simulink model "simple_system_sim"  (R2022a)
settings: Solver=ode45  StartTime=0.0  StopTime=15.0  RelTol=1e-3
values from neighbouring files (symbols this model uses):
  J = 1/4*m*R^2+1/3*m*l^2    (= 0.333958333333)    [simple_system.m]
  Kpp = wcp    (= 31.4159265359)    [simple_system.m]
  Kpv = wcv/mu    (= 104.916104661)    [simple_system.m]
  L = 30    [simple_system.m]
  l = 1.0    (= 1)    [simple_system.m]
  m = 1.0    (= 1)    [simple_system.m]
  Tff = 1/(wff*2*pi)    (= 0.00318309886184)    [simple_system.m]
  Tiv = 1/(0.1*wcv)    (= 0.0318309886184)    [simple_system.m]
  Tlpf = 1/(wlpf*2*pi)    (= 0.0318309886184)    [simple_system.m]
libraries: simulink x6
settings Model: Creator=ale  LastModifiedBy=ale

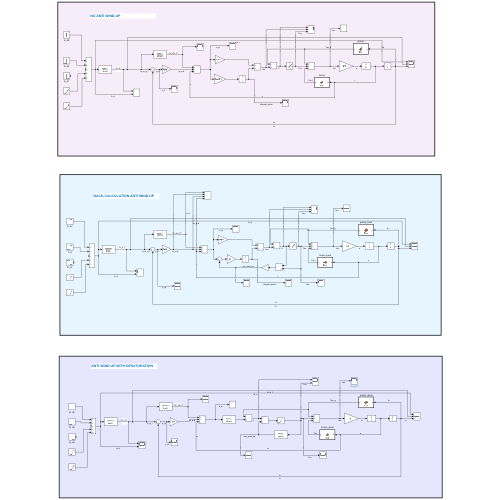
[thumbnail: Simulink's stored preview of the top-level diagram]
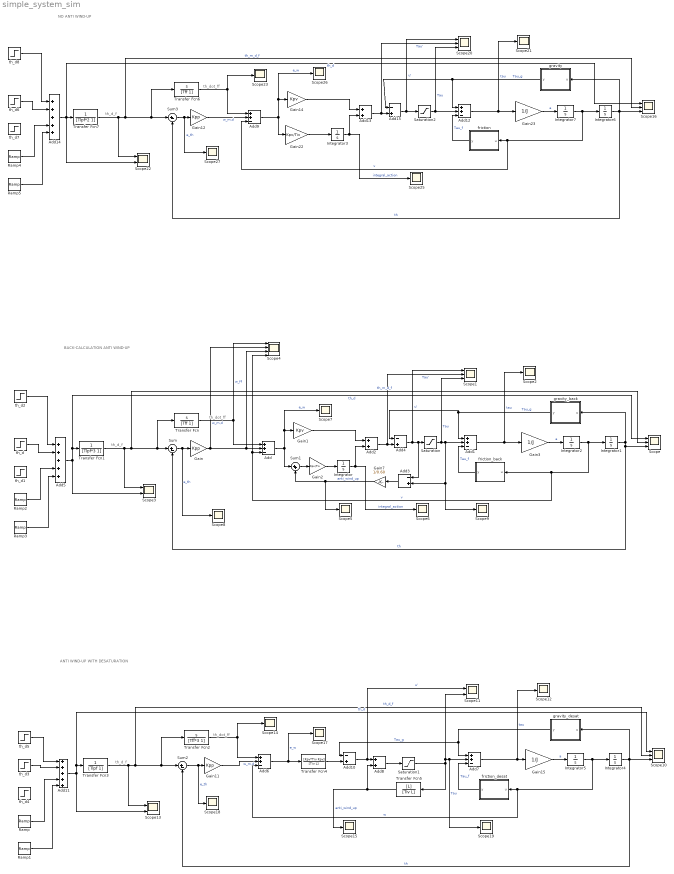
== system simple_system_sim ==
  note: BACK-CALCULATION ANTI WIND-UP
  note: th_dot_ff
  note: th_d_f
  note: th_dot_ff
  note: th_d_f
  note: ANTI WIND-UP WITH DESATURATION
  note: th_d_f
  note: th_dot_ff
  note: NO ANTI WIND-UP
  Add{,1,6..7,9,12} (6 alike) : Sum  Inputs=++-
  Add{3..4,10,15} (4 alike) : Sum  Inputs=-+
  Add11 : Sum  Inputs=+++++
  Add13 : Sum
  Add14 : Sum  Inputs=+++++
  Add2 : Sum
  Add5 : Sum  Inputs=+++++
  Add8 : Sum
  Gain : Gain  Gain=Kpp
  Gain1 : Gain  Gain=Kpv
  Gain11 : Gain  Gain=Kpp
  Gain12 : Gain  Gain=Kpp
  Gain14 : Gain  Gain=Kpv
  Gain15 : Gain  Gain=1/J
  Gain2 : Gain  Gain=Kpv/Tiv
  Gain22 : Gain  Gain=Kpv/Tiv
  Gain23 : Gain  Gain=1/J
  Gain3 : Gain  Gain=1/J
  Gain7 : Gain  Gain=1/0.60
  Integrator{,1..7} (8 alike) : Integrator
  Ramp : simulink/Sources/Ramp  slope=-pi/2  start=6  InitialOutput=0
  Ramp1 : simulink/Sources/Ramp  slope=+pi/2  start=7  InitialOutput=0
  Ramp2 : simulink/Sources/Ramp  slope=-pi/2  start=6  InitialOutput=0
  Ramp3 : simulink/Sources/Ramp  slope=+pi/2  start=7  InitialOutput=0
  Ramp4 : simulink/Sources/Ramp  slope=-pi/2  start=6  InitialOutput=0
  Ramp5 : simulink/Sources/Ramp  slope=+pi/2  start=7  InitialOutput=0
  Saturation : Saturate  UpperLimit=6  LowerLimit=-6
  Saturation1 : Saturate  UpperLimit=6  LowerLimit=-6
  Saturation2 : Saturate  UpperLimit=6  LowerLimit=-6
  Scope{,1,10,16,20} (5 alike) : Scope  NumInputPorts=3
  Scope{3,11,13,22} (4 alike) : Scope  NumInputPorts=2
  Scope{2,5..9,12,14..15,17..19,21,23,25..27} (17 alike) : Scope
  Scope4 : Scope  NumInputPorts=4
  Sum : Sum  Inputs=|+-
  Sum1 : Sum  Inputs=|++
  Sum2 : Sum  Inputs=|+-
  Sum3 : Sum  Inputs=|+-
  Transfer Fcn : TransferFcn  Numerator=[1 0]  Denominator=[Tff 1]
  Transfer Fcn1 : TransferFcn  Denominator=[Tlpf*3 1]
  Transfer Fcn2 : TransferFcn  Numerator=[1 0]  Denominator=[Tff*3 1]
  Transfer Fcn3 : TransferFcn  Denominator=[Tlpf 1]
  Transfer Fcn4 : TransferFcn  Numerator=[Kpv*Tiv Kpv]  Denominator=[Tiv L]
  Transfer Fcn5 : TransferFcn  Numerator=[L]  Denominator=[Tiv L]
  Transfer Fcn6 : TransferFcn  Numerator=[1 0]  Denominator=[Tff 1]
  Transfer Fcn7 : TransferFcn  Denominator=[Tlpf*2 1]
  friction : MATLAB Function  TreatAsAtomicUnit=on
  friction_back : MATLAB Function  TreatAsAtomicUnit=on
  friction_desat : MATLAB Function  TreatAsAtomicUnit=on
  gravity : MATLAB Function  TreatAsAtomicUnit=on
  gravity_back : MATLAB Function  TreatAsAtomicUnit=on
  gravity_desat : MATLAB Function  TreatAsAtomicUnit=on
  th_d : Step  After=pi/18  SampleTime=0
  th_d1 : Step  Time=6  After=-pi/2  SampleTime=0
  th_d2 : Step  Time=3  After=pi/18  SampleTime=0
  th_d3 : Step  After=pi/18  SampleTime=0
  th_d4 : Step  Time=6  After=-pi/2  SampleTime=1
  th_d5 : Step  Time=3  After=pi/18  SampleTime=0
  th_d6 : Step  After=pi/18  SampleTime=0
  th_d7 : Step  Time=6  After=-pi/2  SampleTime=0
  th_d8 : Step  Time=3  After=pi/18  SampleTime=0
  wires:
  Sum/1 -> Gain/1, Scope8/1  "e_th"
  Gain1/1 -> Add2/1
  Integrator/1 -> Add2/2, Scope6/1  "integral_action"
  Add/1 -> Sum1/1, Gain1/1, Scope7/1  "e_w"
  Add2/1 -> Add4/2, Scope1/2  "Tau'"
  Integrator1/1 -> Sum/2, Scope/3, gravity_back/1(u)  "th"
  Gain3/1 -> Integrator2/1  "a"
  Integrator2/1 -> friction_back/1(u), Add/3, Scope4/4, Integrator1/1  "v"
  gravity_back/1(y) -> Add4/1, Add1/1  "Tau_g"
  Transfer Fcn1/1 -> Scope3/1, Transfer Fcn/1, Sum/1, Scope/2  "th_m_d_f"
  Saturation/1 -> Scope9/1, Add3/2, Add1/2, Scope1/3  "Tau"
  Add3/1 -> Gain7/1
  Gain7/1 -> Scope5/1, Sum1/2  "anti_wind_up"
  Add1/1 -> Gain3/1, Scope2/1  "tau"
  Transfer Fcn/1 -> Add/1, Scope4/1  "w_ff"
  Add4/1 -> Scope1/1, Add3/1, Saturation/1  "u'"
  Add5/1 -> Scope3/2, Scope/1, Transfer Fcn1/1  "th_d"
  th_d2/1 -> Add5/1
  th_d/1 -> Add5/2
  Integrator4/1 -> Sum2/2, Scope10/3, gravity_desat/1(u)  "th"
  gravity_desat/1(y) -> Add7/1, Add10/1  "Tau_g"
  Sum2/1 -> Scope18/1, Gain11/1  "e_th"
  Add11/1 -> Scope10/1, Transfer Fcn3/1, Scope13/2  "th_d"
  th_d5/1 -> Add11/1
  th_d3/1 -> Add11/2
  Gain15/1 -> Integrator5/1  "a"
  Add6/1 -> Transfer Fcn4/1, Scope17/1  "e_w"
  Transfer Fcn2/1 -> Scope14/1, Add6/1
  friction_desat/1(y) -> Add7/3  "Tau_f"
  Transfer Fcn3/1 -> Scope13/1, Transfer Fcn2/1, Sum2/1, Scope10/2  "th_d_f"
  Saturation1/1 -> Transfer Fcn5/1, Scope19/1, Add7/2, Scope11/2  "Tau"
  Gain11/1 -> Add6/2  "w_m,d"
  Transfer Fcn5/1 -> Add8/2, Scope15/1  "anti_wind_up"
  Integrator5/1 -> Add6/3, friction_desat/1(u), Integrator4/1  "w"
  Add7/1 -> Gain15/1, Scope12/1  "tau"
  Transfer Fcn4/1 -> Add10/2
  Add10/1 -> Scope11/1, Add8/1  "u'"
  Add8/1 -> Saturation1/1
  friction_back/1(y) -> Add1/3  "Tau_f"
  Saturation2/1 -> Add12/2, Scope20/3  "Tau"
  Add13/1 -> Add15/2, Scope20/2  "Tau'"
  Gain14/1 -> Add13/1
  Add14/1 -> Scope16/1, Scope22/2, Transfer Fcn7/1  "th_d"
  Gain12/1 -> Add9/2  "w_m,d"
  Gain23/1 -> Integrator7/1  "a"
  Transfer Fcn6/1 -> Scope23/1, Add9/1
  Add15/1 -> Scope20/1, Saturation2/1  "u'"
  gravity/1(y) -> Add12/1, Add15/1  "Tau_g"
  friction/1(y) -> Add12/3  "Tau_f"
  Sum3/1 -> Scope27/1, Gain12/1  "e_th"
  Integrator6/1 -> Sum3/2, Scope16/3, gravity/1(u)  "th"
  Gain22/1 -> Integrator3/1
  Integrator7/1 -> Add9/3, friction/1(u), Integrator6/1  "v"
  Integrator3/1 -> Add13/2, Scope25/1  "integral_action"
  Add12/1 -> Gain23/1, Scope21/1  "tau"
  Add9/1 -> Gain14/1, Scope26/1, Gain22/1  "e_w"
  Transfer Fcn7/1 -> Scope22/1, Transfer Fcn6/1, Sum3/1, Scope16/2  "th_m_d_f"
  Ramp/1 -> Add11/4
  Ramp1/1 -> Add11/5
  Sum1/1 -> Gain2/1
  Gain2/1 -> Integrator/1
  Ramp3/1 -> Add5/5
  Ramp2/1 -> Add5/4
  Gain/1 -> Scope4/3, Add/2, Scope4/2  "w_m,d"
  th_d8/1 -> Add14/1
  th_d6/1 -> Add14/2
  Ramp5/1 -> Add14/5
  Ramp4/1 -> Add14/4

== matlab function simple_system_sim/gravity_back ==
  data: u input; y output; m parameter; l parameter
function y = fcn(u,m, l)
y = m*9.81*l/2*sin(u);

== matlab function simple_system_sim/gravity_desat ==
  data: u input; y output; m parameter; l parameter
function y = fcn(u,m, l)
y = m*9.81*l/2*sin(u);

== matlab function simple_system_sim/friction_desat ==
  data: u input; y output
function y = fcn(u)
y = 0.1*u + 0.4*sign(u);

== matlab function simple_system_sim/gravity ==
  data: u input; y output; m parameter; l parameter
function y = fcn(u,m, l)
y = m*9.81*l/2*sin(u);

== matlab function simple_system_sim/friction ==
  data: u input; y output
function y = fcn(u)
y = 0.1*u + 0.4*sign(u);

== matlab function simple_system_sim/friction_back ==
  data: u input; y output
function y = fcn(u)
y = 0.1*u + 0.4*sign(u);
